simulink model "clarke_park"  (R2023b)
settings: Solver=VariableStepAuto  StartTime=0.0  StopTime=0.1  MaxStep=1e-4  RelTol=1e-3
libraries: spsabctoAlphaBetaZeroLib x1, spsabctodq0Lib x1, spsPLL3phLib x1, spsAlphaBetaZerotodq0Lib x1
settings Model: Creator=Vissu  LastModifiedBy=Vissu

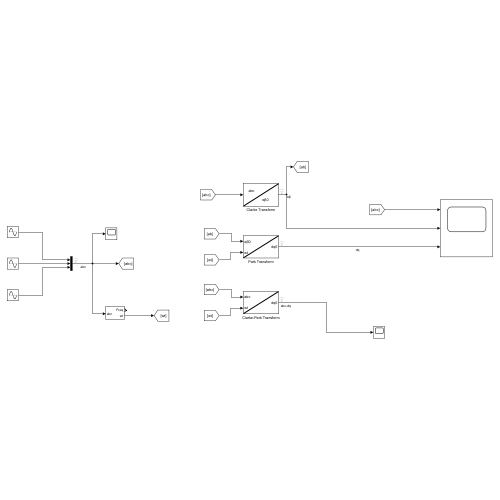
[thumbnail: Simulink's stored preview of the top-level diagram]
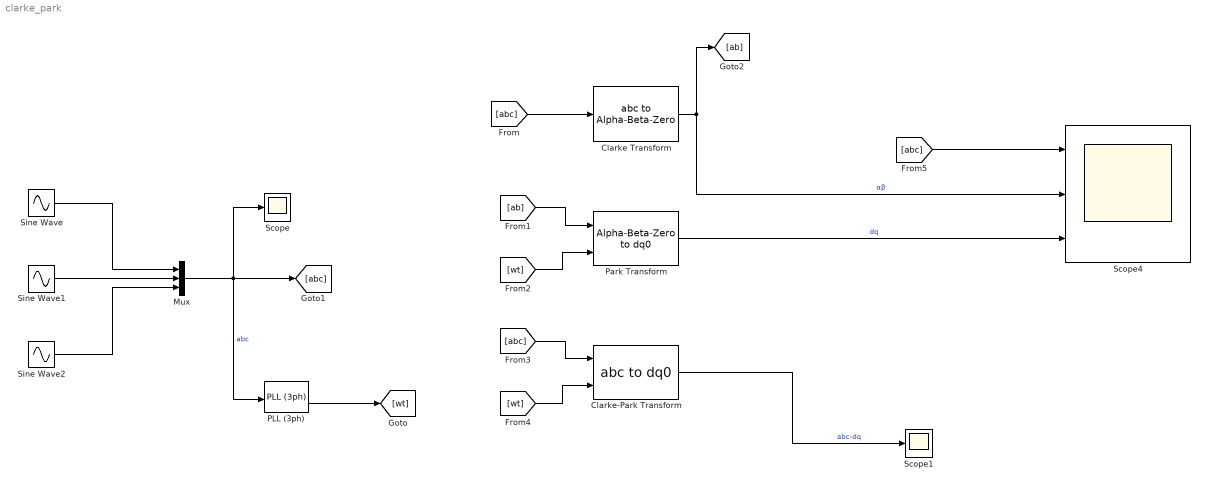
== system clarke_park ==
  Clarke Transform : spsabctoAlphaBetaZeroLib/abc to Alpha-Beta-Zero
  Clarke-Park Transform : spsabctodq0Lib/abc to dq0  Alignment=90 degrees behind phase A axis
  Mux : Mux  Inputs=3
  PLL (3ph) : spsPLL3phLib/PLL (3ph)  Fmin=45  Par_Init=[0, 50]  ParK=[180, 3200, 1]  TcD=1e-4  MaxRateChangeFreq=12  FilterCutOffFreq=25  Ts=0  AGC=on
  Park Transform : spsAlphaBetaZerotodq0Lib/Alpha-Beta-Zero to dq0  Alignment=90 degrees behind phase A axis
  Scope : Scope
  Scope1 : Scope
  Scope4 : Scope  NumInputPorts=3
  Sine Wave : Sin  Frequency=2*pi*50  SampleTime=0
  Sine Wave1 : Sin  Frequency=2*pi*50  Phase=-120*(pi/180)  SampleTime=0
  Sine Wave2 : Sin  Frequency=2*pi*50  Phase=120*(pi/180)  SampleTime=0
  wires:
  Sine Wave/1 -> Mux/1
  Sine Wave1/1 -> Mux/2
  Sine Wave2/1 -> Mux/3
  Mux/1 -> PLL (3ph)/1, [abc], Scope/1  "abc"
  PLL (3ph)/2 -> [wt]
  [abc] -> Clarke Transform/1
  Clarke Transform/1 -> Scope4/2, [ab]  "αβ"
  [ab] -> Park Transform/1
  [wt] -> Park Transform/2
  Park Transform/1 -> Scope4/3  "dq"
  [abc] -> Clarke-Park Transform/1
  [wt] -> Clarke-Park Transform/2
  Clarke-Park Transform/1 -> Scope1/1  "abc-dq"
  [abc] -> Scope4/1
